simulink model "modelo_fanplate"  (R2023b)
settings: Solver=VariableStepAuto  StartTime=0.0  StopTime=30  RelTol=1e-3
values from neighbouring files (symbols this model uses):
  A1 = -0.036    [modelo_fan_plate.m]
  A2 = 0.085    [modelo_fan_plate.m]
  Fg = m*g    (= 1.10853)    [modelo_fan_plate.m]
  G1 = 0    [modelo_fan_plate.m]
  Jm = 4.079e-3    (= 0.004079)    [modelo_fan_plate.m]
  Jp = 5.23e-4    (= 0.000523)    [modelo_fan_plate.m]
  Ka = 1/Kw    (= 30.303030303)    [modelo_fan_plate.m]
  Kap = 3.11e-6    (= 3.11e-06)    [modelo_fan_plate.m]
  KD = Pu/8    (= 0.0105625)    [modelo_fan_plate.m]
  KI = Pu/2    (= 0.04225)    [modelo_fan_plate.m]
  KP = 0.6*Kcu    (= 360)    [modelo_fan_plate.m]
  Kw = 0.033    [modelo_fan_plate.m]
  L_m = 0.157    [modelo_fan_plate.m]
  La = 1e-3    (= 0.001)    [modelo_fan_plate.m]
  Pos_sat_under = 0*pi/180    (= 0)    [modelo_fan_plate.m]
  Pos_sat_upper = 90*pi/180    (= 1.57079632679)    [modelo_fan_plate.m]
  Ra = 10    [modelo_fan_plate.m]
  V_max = 16    [modelo_fan_plate.m]
  V_min = 0.0    (= 0)    [modelo_fan_plate.m]
libraries: slpidlib x1
settings Model: Creator=hugo  LastModifiedBy=hugo

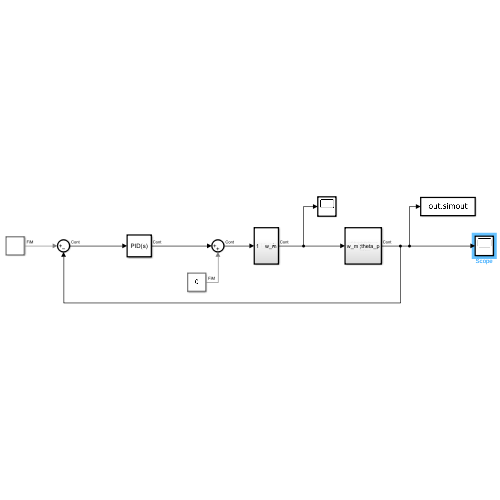
[thumbnail: Simulink's stored preview of the top-level diagram]
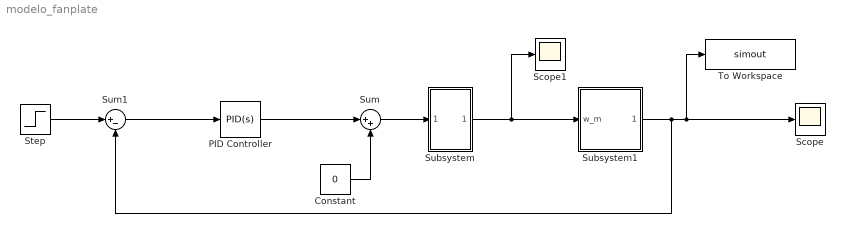
== system modelo_fanplate ==
  Constant : Constant  Value=0  SampleTime=0
  PID Controller : slpidlib/PID Controller  Controller=PID  Form=Parallel  TimeDomain=Continuous-time  UseExternalTs=off  SampleTime=-1  IntegratorMethod=Forward Euler  FilterMethod=Forward Euler  ControllerParametersSource=internal  P=KP  I=KI  UseKiTs=off  D=KD  N=100  UseFilter=on  TunerSelectOption=Transfer Function Based (PID Tuner App)  InitialConditionSource=internal  InitialConditionForIntegrator=0  InitialConditionForFilter=0  DifferentiatorICPrevScaledInput=0  ExternalReset=none  TrackingMode=off  Kt=1  LimitOutput=off  SatLimitsSource=internal  UpperSaturationLimit=inf  LowerSaturationLimit=-inf  LinearizeAsGain=on  AntiWindupMode=none  Kb=1  LimitIntegrator=off  UpperIntegratorSaturationLimit=inf  LowerIntegratorSaturationLimit=-inf  POutMin=[]  POutMax=[]  IOutMin=[]  IOutMax=[]  DOutMin=[]  DOutMax=[]  NOutMin=[]  NOutMax=[]  SumOutMin=[]  SumOutMax=[]  SaturationOutMin=[]  SaturationOutMax=[]  PParamMin=[]  PParamMax=[]  IParamMin=[]  IParamMax=[]  DParamMin=[]  DParamMax=[]  NParamMin=[]  NParamMax=[]  KbParamMin=[]  KbParamMax=[]  KtParamMin=[]  KtParamMax=[]  KbOutMin=[]  KbOutMax=[]  KtOutMin=[]  KtOutMax=[]  IntegratorOutMin=[]  IntegratorOutMax=[]  FilterOutMin=[]  FilterOutMax=[]  SumI1OutMin=[]  SumI1OutMax=[]  SumI2OutMin=[]  SumI2OutMax=[]  SumI3OutMin=[]  SumI3OutMax=[]  SumI4OutMin=[]  SumI4OutMax=[]  SumDOutMin=[]  SumDOutMax=[]  DifferentiatorOutMin=[]  DifferentiatorOutMax=[]  FilterDiffOutCoefMin=[]  FilterDiffOutCoefMax=[]  ReciprocalOutMin=[]  ReciprocalOutMax=[]  SumDenOutMin=[]  SumDenOutMax=[]  SumNumOutMin=[]  SumNumOutMax=[]  DivideOutMin=[]  DivideOutMax=[]  UdiffTsProdOutMin=[]  UdiffTsProdOutMax=[]  NTsProdOutMin=[]  NTsProdOutMax=[]  UintegralTsProdOutMin=[]  UintegralTsProdOutMax=[]  UngainTsProdOutMin=[]  UngainTsProdOutMax=[]  ClampingZeroOutDataTypeStr=Inherit: Inherit via back propagation  ClampingZeroOutMin=[]  ClampingZeroOutMax=[]  FilterDenConstantOutDataTypeStr=Inherit: Inherit via back propagation  FilterDenConstantOutMin=[]  FilterDenConstantOutMax=[]  PCopyOutDataTypeStr=Inherit: Inherit via back propagation  PCopyOutMin=[]  PCopyOutMax=[]  NCopyOutDataTypeStr=Inherit: Inherit via back propagation  NCopyOutMin=[]  NCopyOutMax=[]  IntegratorContinuousStateAttributes=''  IntegratorStateMustResolveToSignalObject=off  IntegratorRTWStateStorageClass=Auto  FilterContinuousStateAttributes=''  FilterStateMustResolveToSignalObject=off  FilterRTWStateStorageClass=Auto  ParallelPVariant=InternalParameters  IdealPVariant=Disabled  IVariant=InternalParameters  DVariant=InternalParameters  IntegratorVariant=Continuous  SatVariant=Disabled  AWVariant=Passthrough  PCopyVariant=Disabled  TRVariant=Disabled  FdbkBlocksVariant=Forward  IdealPFdbkVariant=Disabled  SatFdbkVariant=Disabled  DerivativeFilterVariant=ContFilter  NVariant=InternalParameters  NCopyVariant=Disabled  FilterICVariant=InternalICsFilter  IntegratorICVariant=InternalICs  ExternalResetVariant=Disabled  TRSumVariant=Passthrough  SumFdbkVariant=Disabled  SumVariant=Sum_PID  TsampFilterVariant=InternalTs  TsampNgainVariant=Passthrough  TsampIntegralVariant=Disabled_SignalSpec  ExternalSaturationOutDataTypeStr=Inherit: Same as second input
  Scope : Scope
  Scope1 : Scope
  Step : Step  Time=0  After=deg2rad(50)  SampleTime=0
  Subsystem : Subsystem
  Subsystem1 : Subsystem
  Sum : Sum  Inputs=|++
  Sum1 : Sum  Inputs=|+-
  To Workspace : ToWorkspace  VariableName=simout  SaveFormat=Timeseries  SampleTime=-1
  wires:
  Subsystem1/1(theta_p) -> Sum1/2, To Workspace/1, Scope/1
  Subsystem/1(w_m) -> Scope1/1, Subsystem1/1(w_m)
  Sum/1 -> Subsystem/1(In1)
  Step/1 -> Sum1/1
  Constant/1 -> Sum/2
  PID Controller/1 -> Sum/1
  Sum1/1 -> PID Controller/1

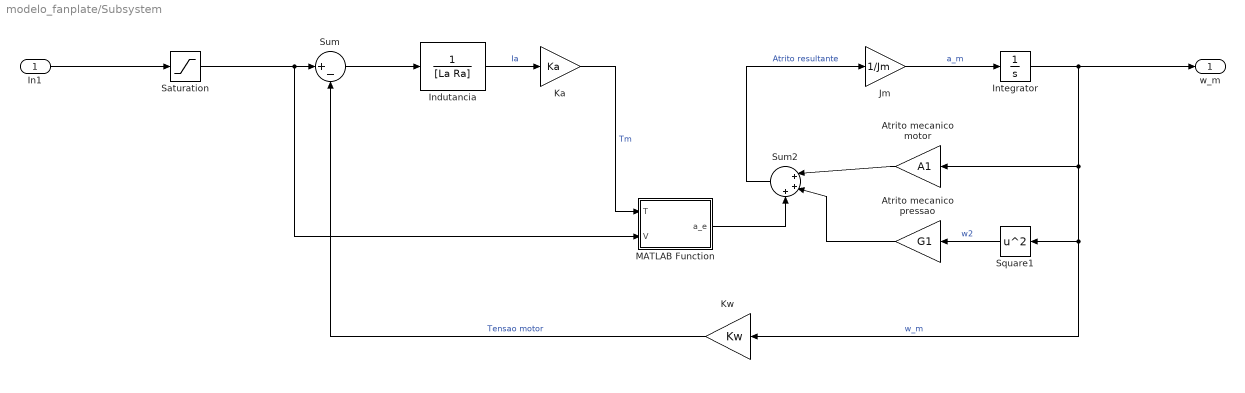
== system modelo_fanplate/Subsystem ==
  In1 : Inport
  Atrito mecanico motor : Gain  Gain=A1
  Atrito mecanico pressao : Gain  Gain=G1
  Indutancia : TransferFcn  Denominator=[La Ra]
  Integrator : Integrator
  Jm : Gain  Gain=1/Jm
  Ka : Gain  Gain=Ka
  Kw : Gain  Gain=Kw
  MATLAB Function : MATLAB Function  TreatAsAtomicUnit=on
  Saturation : Saturate  UpperLimit=V_max  LowerLimit=V_min
  Square1 : Math  Operator=square
  Sum : Sum  Inputs=|+-
  Sum2 : Sum  Inputs=|+++
  w_m : Outport
  wires:
  Kw/1 -> Sum/2  "Tensao motor"
  Jm/1 -> Integrator/1  "a_m"
  Atrito mecanico motor/1 -> Sum2/1
  In1/1 -> Saturation/1
  MATLAB Function/1(a_e) -> Sum2/3
  Indutancia/1 -> Ka/1  "Ia"
  Saturation/1 -> MATLAB Function/2(V), Sum/1
  Atrito mecanico pressao/1 -> Sum2/2
  Square1/1 -> Atrito mecanico pressao/1  "w2"
  Sum2/1 -> Jm/1  "Atrito resultante"
  Sum/1 -> Indutancia/1
  Ka/1 -> MATLAB Function/1(T)  "Tm"
  Integrator/1 -> w_m/1, Square1/1, Kw/1, Atrito mecanico motor/1  "w_m"

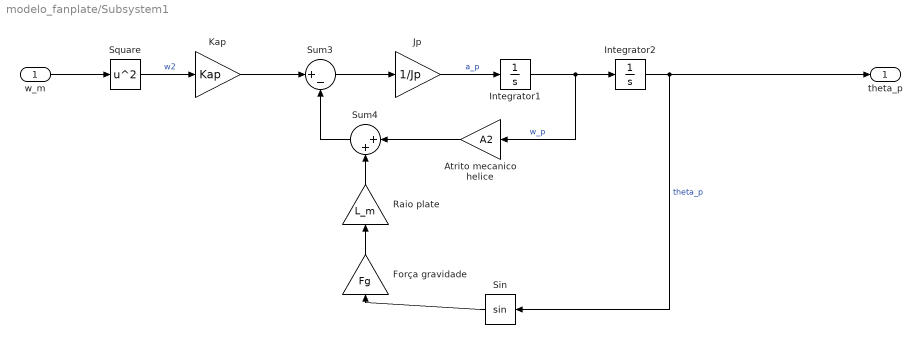
== system modelo_fanplate/Subsystem1 ==
  w_m : Inport
  Atrito mecanico helice : Gain  Gain=A2
  Força gravidade : Gain  Gain=Fg
  Integrator1 : Integrator
  Integrator2 : Integrator  LimitOutput=on  UpperSaturationLimit=Pos_sat_upper  LowerSaturationLimit=Pos_sat_under
  Jp : Gain  Gain=1/Jp
  Kap : Gain  Gain=Kap
  Raio plate : Gain  Gain=L_m
  Sin : Trigonometry
  Square : Math  Operator=square
  Sum3 : Sum  Inputs=|+-
  Sum4 : Sum  Inputs=|++
  theta_p : Outport
  wires:
  Jp/1 -> Integrator1/1  "a_p"
  Raio plate/1 -> Sum4/2
  Força gravidade/1 -> Raio plate/1
  Sum4/1 -> Sum3/2
  Kap/1 -> Sum3/1
  Atrito mecanico helice/1 -> Sum4/1
  Integrator1/1 -> Atrito mecanico helice/1, Integrator2/1  "w_p"
  Sum3/1 -> Jp/1
  Sin/1 -> Força gravidade/1
  w_m/1 -> Square/1
  Square/1 -> Kap/1  "w2"
  Integrator2/1 -> theta_p/1, Sin/1  "theta_p"

== matlab function modelo_fanplate/Subsystem/MATLAB Function ==
  data: T input; a_e output; V input
function a_e = atrito_e(T,V)

if V <3
    a_e = 0;
else
    a_e = T;
end

end
